simulink subsystem "Physical_system"  (R2020a)
settings: Solver=VariableStepAuto  StartTime=0.0  StopTime=10.0  RelTol=1e-3
libraries: aerolibgravity2 x2, aerolibconvert2 x1
settings Model: Creator=decla  LastModifiedBy=decla

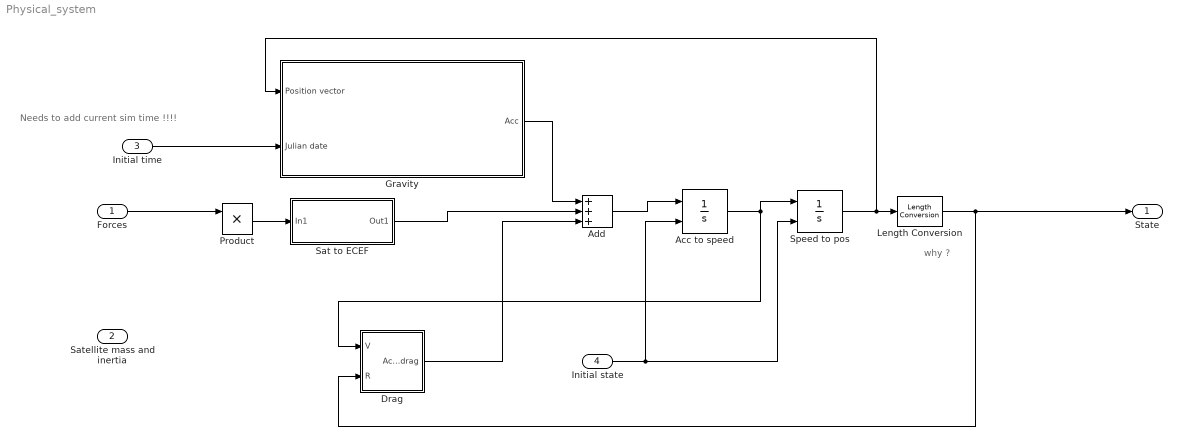
== system Physical_system ==
  note: why ?
  note: Needs to add current sim time !!!!
  Forces : Inport
  Satellite mass and inertia : Inport  Port=2
  Initial time : Inport  Port=3
  Initial state : Inport  Port=4
  Acc to speed : Integrator  InitialConditionSource=external  InitialCondition=[-2871.828;-5954.63;3774.64]
  Add : Sum  Inputs=+++
  Drag : Subsystem
  Gravity : Subsystem
  Length Conversion : aerolibconvert2/Length Conversion  IU=m  OU=km
  Product : Product
  Sat to ECEF : Subsystem
  Speed to pos : Integrator  InitialConditionSource=external  InitialCondition=[2383.89e3;2594.67e3;5906.12e3]
  State : Outport
  wires:
  Drag/1(Acc_drag) -> Add/3
  Add/1 -> Acc to speed/1
  Gravity/1(Acc) -> Add/1
  Speed to pos/1 -> Gravity/1(Position vector), Length Conversion/1
  Acc to speed/1 -> Speed to pos/1, Drag/1(V)
  Length Conversion/1 -> Drag/2(R), State/1
  Sat to ECEF/1(Out1) -> Add/2
  Forces/1 -> Product/1
  Product/1 -> Sat to ECEF/1(In1)
  Initial time/1 -> Gravity/2(Julian date)
  Initial state/1 -> Acc to speed/2, Speed to pos/2

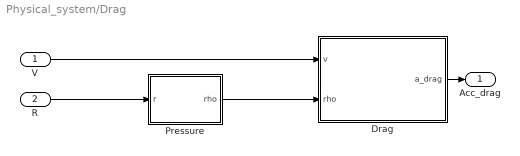
== system Physical_system/Drag ==
  V : Inport
  R : Inport  Port=2
  Drag : MATLAB Function  TreatAsAtomicUnit=on
  Pressure : MATLAB Function  TreatAsAtomicUnit=on
  Acc_drag : Outport
  wires:
  R/1 -> Pressure/1(r)
  V/1 -> Drag/1(v)
  Drag/1(a_drag) -> Acc_drag/1
  Pressure/1(rho) -> Drag/2(rho)

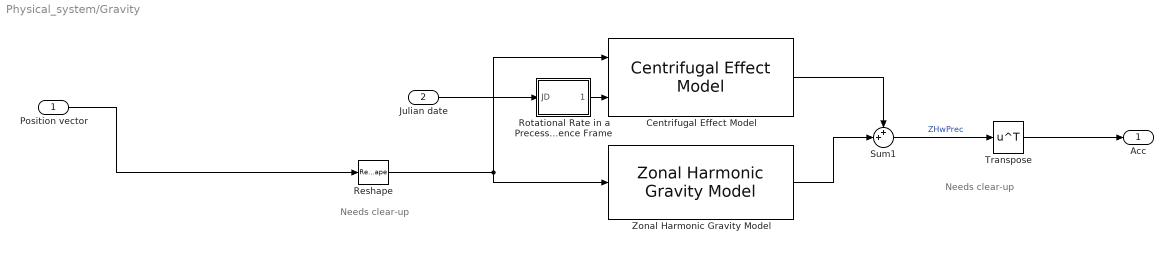
== system Physical_system/Gravity ==
  note: Needs clear-up
  note: Needs clear-up
  Position vector : Inport
  Julian date : Inport  Port=2
  Centrifugal Effect Model : aerolibgravity2/Centrifugal Effect Model  ptype=Custom  omega=7.2921150e-005  rate_loc=on
      settings: SourceProductBaseCode=AE
  Reshape : Reshape  OutputDimensionality=Row vector (2-D)
  Rotational Rate in a Precessing Reference Frame : Subsystem
  Sum1 : Sum  Inputs=++|
  Transpose : Math  Operator=transpose  SaturateOnIntegerOverflow=on
  Zonal Harmonic Gravity Model : aerolibgravity2/Zonal Harmonic Gravity Model  units=Metric (MKS)  degree=4  action=Warning  ptype=Earth  R=6378136.3  GM=398600441500000  jvalue=[1.0826269e-03 -2.5323000e-06 -1.6204000e-06]
      settings: SourceProductBaseCode=AE
  Acc : Outport
  wires:
  Transpose/1 -> Acc/1
  Sum1/1 -> Transpose/1  "ZHwPrec"
  Centrifugal Effect Model/1 -> Sum1/1
  Zonal Harmonic Gravity Model/1 -> Sum1/2
  Julian date/1 -> Rotational Rate in a Precessing Reference Frame/1(JD)
  Position vector/1 -> Reshape/1
  Rotational Rate in a Precessing Reference Frame/1(omega) -> Centrifugal Effect Model/2
  Reshape/1 -> Zonal Harmonic Gravity Model/1, Centrifugal Effect Model/1

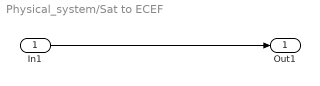
== system Physical_system/Sat to ECEF ==
  In1 : Inport
  Out1 : Outport
  wires:
  In1/1 -> Out1/1

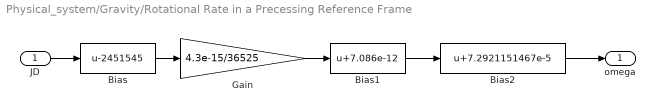
== system Physical_system/Gravity/Rotational Rate in a Precessing Reference Frame ==
  JD : Inport
  Bias : Bias  Bias=-2451545
  Bias1 : Bias  Bias=7.086e-12
  Bias2 : Bias  Bias=7.2921151467e-5
  Gain : Gain  Gain=4.3e-15/36525
  omega : Outport  VectorParamsAs1DForOutWhenUnconnected=off
  wires:
  Bias2/1 -> omega/1
  Bias1/1 -> Bias2/1
  Gain/1 -> Bias1/1
  Bias/1 -> Gain/1
  JD/1 -> Bias/1

== matlab function Physical_system/Drag/Pressure ==
  data: r input; rho output
function rho = fcn(r)
alt = norm(r);
A = 1.140564e-10;
B = -2.130756e-7;
C = 1.570562e-4;
D = -0.07029296;
E = -12.89844;

rho = exp(A*alt^4 + B*alt^3 + C*alt^2 + D*alt + E);

== matlab function Physical_system/Drag/Drag ==
  data: v input; a_drag output; rho input
function a_drag = fcn(v, rho)
area = 100e-4;
mass = 3;
V = norm(v);
Cd = 1.05;

a_drag = -0.5*Cd*(area/mass)*rho*V^2;
